simulink model "ECE545HW5"  (R2017a)
settings: Solver=VariableStepAuto  StartTime=0.0  StopTime=10.0  RelTol=1e-3
settings Model: Creator=clarke6  LastModifiedBy=clarke6

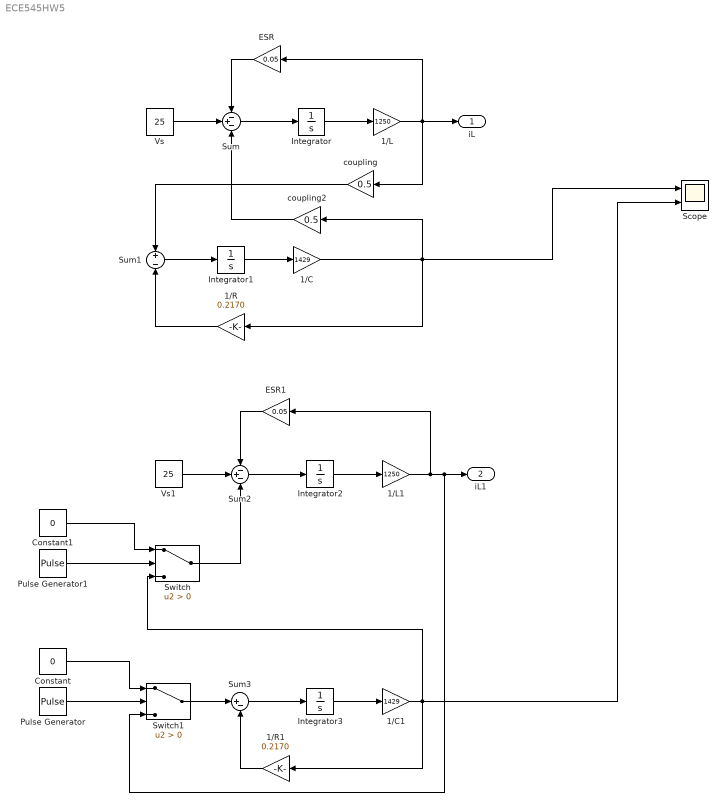
== system ECE545HW5 ==
  1/C : Gain  Gain=1429
  1/C1 : Gain  Gain=1429
  1/L : Gain  Gain=1250
  1/L1 : Gain  Gain=1250
  1/R : Gain  Gain=0.2170
  1/R1 : Gain  Gain=0.2170
  Constant : Constant  Value=0
  Constant1 : Constant  Value=0
  ESR : Gain  Gain=0.05
  ESR1 : Gain  Gain=0.05
  Integrator{,1..3} (4 alike) : Integrator
  Pulse Generator : DiscretePulseGenerator  PulseType=Time based  Period=0.00005  PulseWidth=50
  Pulse Generator1 : DiscretePulseGenerator  PulseType=Time based  Period=0.00005  PulseWidth=50
  Scope : Scope  NumInputPorts=2
  Sum : Sum  Inputs=-+-
  Sum1 : Sum  Inputs=+|-
  Sum2 : Sum  Inputs=-+-
  Sum3 : Sum  Inputs=|+-
  Switch : Switch  Criteria=u2 > Threshold
  Switch1 : Switch  Criteria=u2 > Threshold
  Vs : Constant  Value=25
  Vs1 : Constant  Value=25
  coupling : Gain  Gain=0.5
  coupling2 : Gain  Gain=0.5
  iL : Outport
  iL1 : Outport  Port=2
  wires:
  Sum/1 -> Integrator/1
  Integrator/1 -> 1/L/1
  1/L/1 -> iL/1, coupling/1, ESR/1
  Vs/1 -> Sum/2
  ESR/1 -> Sum/1
  coupling/1 -> Sum1/1
  Sum1/1 -> Integrator1/1
  Integrator1/1 -> 1/C/1
  1/C/1 -> Scope/1, coupling2/1, 1/R/1
  1/R/1 -> Sum1/2
  coupling2/1 -> Sum/3
  ESR1/1 -> Sum2/1
  Sum2/1 -> Integrator2/1
  1/L1/1 -> Switch1/3, iL1/1, ESR1/1
  Vs1/1 -> Sum2/2
  Integrator2/1 -> 1/L1/1
  Constant1/1 -> Switch/1
  Pulse Generator1/1 -> Switch/2
  Switch/1 -> Sum2/3
  Constant/1 -> Switch1/1
  Pulse Generator/1 -> Switch1/2
  Switch1/1 -> Sum3/1
  Sum3/1 -> Integrator3/1
  Integrator3/1 -> 1/C1/1
  1/C1/1 -> Scope/2, 1/R1/1, Switch/3
  1/R1/1 -> Sum3/2
